simulink model "Virtual_Differential"  (R2019b)
settings: Solver=VariableStepAuto  StartTime=0.0  StopTime=30  RelTol=1e-3
undefined symbols (not defined in the file or in its folder): VEH
libraries: vehdynlibsteering x1
settings Model: EnablePacing=on  Creator=alelu  LastModifiedBy=alelu

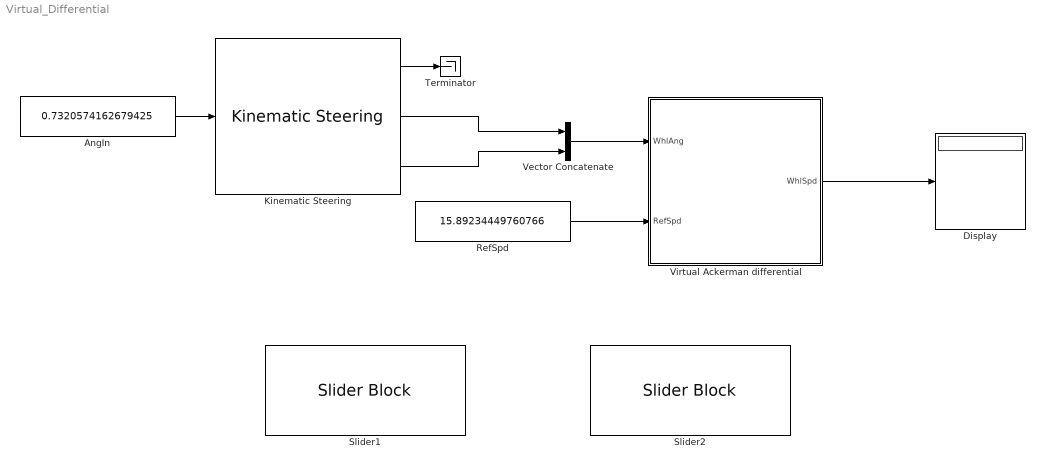
== system Virtual_Differential ==
  AngIn : Constant  Value=0.7320574162679425
  Display : Display
  Kinematic Steering : vehdynlibsteering/Kinematic Steering  StrgType=Ackerman  StrgRatioType=Constant  Loc=Front  NrmlFctr=1  TrckWdth=1.922  WhlBase=VEH.FrontAxlePositionfromCG+VEH.RearAxlePositionfromCG  Db=0  StrgRng=3*pi  StrgAngBpts="[-6.2832   -5.0265   -3.7699   -2.5133   -1.2566         0    1.2566    2.5133    3.7699    5.0265    6.2832]"  StrgRatioTbl=|  StrgRatio=18  StrgArmLngth=0.1  RckCsLngth=0.5  TieRodLngth=0.248128028933392  D=0.2  PnnRadius=0.0057  PnnRadiusTbl="[0.0055    0.0055    0.0056    0.0057    0.0057    0.0057    0.0057    0.0057    0.0056    0.0055    0.0055]"  RodLngth=0.1  ParaArmLngth=0.9  aMode=2
      | [13.5000   13.3750   13.2500   13.1250   13.0000   13.0000   13.0000   13.1250   13.2500   13.3750   13.5000
      | ]
      settings: SourceProductName=Vehicle Dynamics Blockset
  RefSpd : Constant  Value=15.89234449760766
  Slider1 : SliderBlock  ScaleMin=-1  ScaleMax=1  TickInterval=0.5
  Slider2 : SliderBlock  ScaleMin=-8  ScaleMax=40  TickInterval=8
  Terminator : Terminator
  Vector Concatenate : Concatenate
  Virtual Ackerman differential : Subsystem
  wires:
  Virtual Ackerman differential/1(WhlSpd) -> Display/1
  RefSpd/1 -> Virtual Ackerman differential/2(RefSpd)
  Vector Concatenate/1 -> Virtual Ackerman differential/1(WhlAng)
  Kinematic Steering/2 -> Vector Concatenate/1
  Kinematic Steering/3 -> Vector Concatenate/2
  Kinematic Steering/1 -> Terminator/1
  AngIn/1 -> Kinematic Steering/1

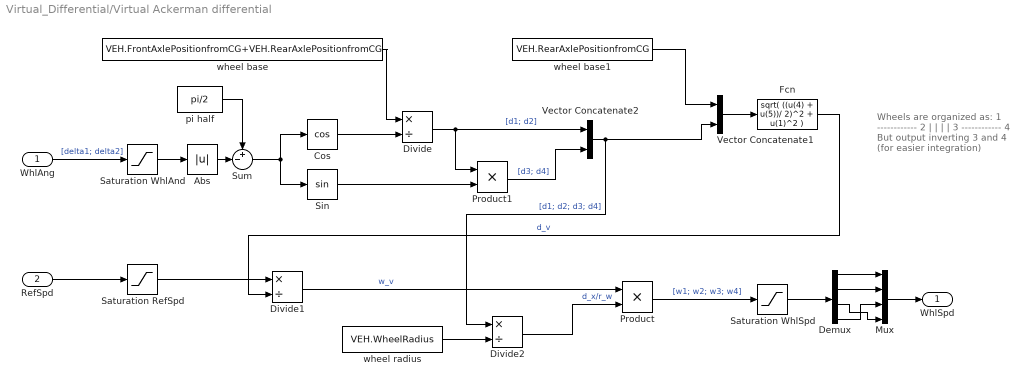
== system Virtual_Differential/Virtual Ackerman differential ==
  note: Wheels are organized as:
      |
      | 1 ------------ 2
      | |
      | |
      | |
      | |
      | 3 ------------ 4
      |
      | But output inverting 3 and 4
      | (for easier integration)
  WhlAng : Inport
  RefSpd : Inport  Port=2
  Abs : Abs
  Cos : Trigonometry  Operator=cos
  Demux : Demux
  Divide : Product  Inputs=*/
  Divide1 : Product  Inputs=*/
  Divide2 : Product  Inputs=*/
  Fcn : Fcn  Expr=sqrt( ((u(4) + u(5))/ 2)^2 + u(1)^2 )
  Mux : Mux
  Product : Product
  Product1 : Product
  Saturation RefSpd : Saturate  UpperLimit=120  LowerLimit=-120
  Saturation WhlAnd : Saturate  UpperLimit=pi*5/12  LowerLimit=-pi*5/12
  Saturation WhlSpd : Saturate  UpperLimit=600  LowerLimit=-600
  Sin : Trigonometry
  Sum : Sum  Inputs=+-|
  Vector Concatenate1 : Concatenate
  Vector Concatenate2 : Concatenate
  pi half : Constant  Value=pi/2
  wheel base : Constant  Value=VEH.FrontAxlePositionfromCG+VEH.RearAxlePositionfromCG
  wheel base1 : Constant  Value=VEH.RearAxlePositionfromCG
  wheel radius : Constant  Value=VEH.WheelRadius
  WhlSpd : Outport
  wires:
  Sin/1 -> Product1/2
  Cos/1 -> Divide/2
  wheel base/1 -> Divide/1
  Divide/1 -> Vector Concatenate2/1, Product1/1  "[d1; d2]"
  Vector Concatenate1/1 -> Fcn/1
  Fcn/1 -> Divide1/2  "d_v"
  Divide1/1 -> Product/1  "w_v"
  Divide2/1 -> Product/2  "d_x/r_w"
  wheel radius/1 -> Divide2/2
  pi half/1 -> Sum/1
  Sum/1 -> Sin/1, Cos/1
  Product1/1 -> Vector Concatenate2/2  "[d3; d4]"
  Vector Concatenate2/1 -> Divide2/1, Vector Concatenate1/2  "[d1; d2; d3; d4]"
  Abs/1 -> Sum/2
  Saturation WhlAnd/1 -> Abs/1
  WhlAng/1 -> Saturation WhlAnd/1  "[delta1; delta2]"
  Saturation RefSpd/1 -> Divide1/1
  RefSpd/1 -> Saturation RefSpd/1
  Product/1 -> Saturation WhlSpd/1  "[w1; w2; w3; w4]"
  Saturation WhlSpd/1 -> Demux/1
  Mux/1 -> WhlSpd/1
  Demux/1 -> Mux/1
  Demux/2 -> Mux/2
  Demux/4 -> Mux/3
  Demux/3 -> Mux/4
  wheel base1/1 -> Vector Concatenate1/1
